simulink model "ThreephaseInverterWithoutLCfilter"  (R2024a)
settings: Solver=VariableStepAuto  StartTime=0.0  StopTime=.1  RelTol=1e-3
libraries: spsIGBTDiodeLib x6, simulink x3, spsVoltageMeasurementLib x3, spsDCVoltageSourceLib x1, spsGroundLib x1, spsSawtoothGeneratorLib x1, spsTHDLib x1, spsThreePhaseParallelRLCBranchLib x1, spsThreePhaseVIMeasurementLib x1, spspowerguiLib x1
settings Model: Creator=farza  LastModifiedBy=farza
settings DataIOCC: ReturnWorkspaceOutputs=off

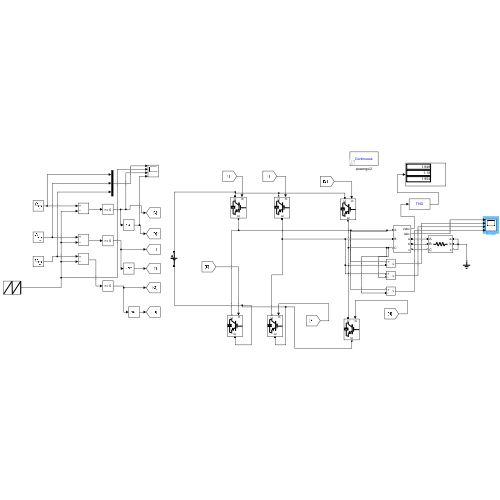
[thumbnail: Simulink's stored preview of the top-level diagram]
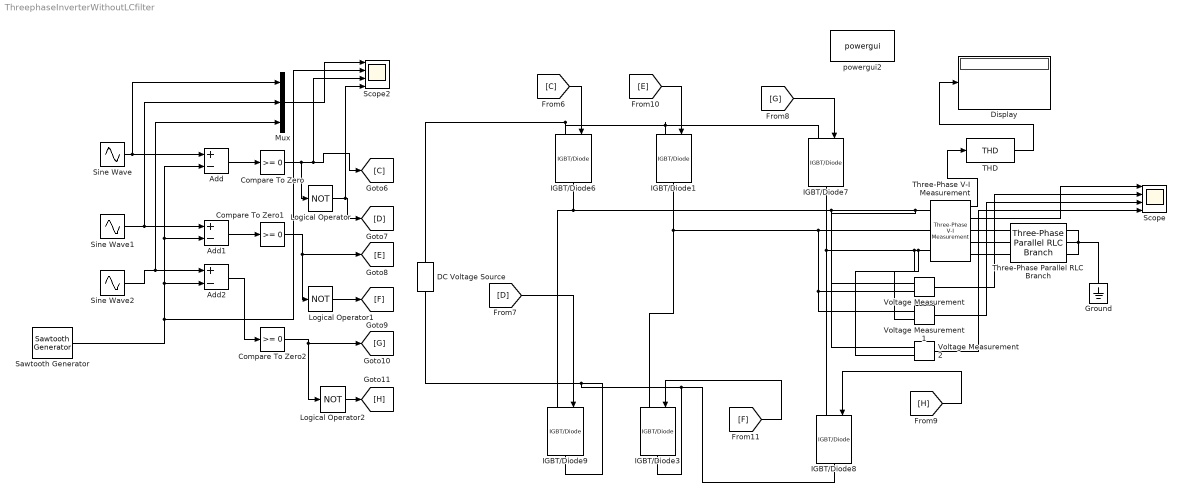
== system ThreephaseInverterWithoutLCfilter ==
  Add : Sum  Inputs=+-
  Add1 : Sum  Inputs=+-
  Add2 : Sum  Inputs=+-
  Compare To Zero : simulink/Logic and Bit Operations/Compare To Zero  relop=>=  OutDataTypeStr=boolean
  Compare To Zero1 : simulink/Logic and Bit Operations/Compare To Zero  relop=>=  OutDataTypeStr=boolean
  Compare To Zero2 : simulink/Logic and Bit Operations/Compare To Zero  relop=>=  OutDataTypeStr=boolean
  DC Voltage Source : spsDCVoltageSourceLib/DC Voltage Source  Amplitude=600  Measurements=None
  Display : Display
  Ground : spsGroundLib/Ground  LConnTagsString=a
  IGBT/Diode{1,3,6..9} (6 alike) : spsIGBTDiodeLib/IGBT//Diode  Ron=1e-3  Rs=1e5  Cs=inf  Measurements=off
  Logical Operator : Logic  Operator=NOT  AllPortsSameDT=off  OutDataTypeStr=boolean
  Logical Operator1 : Logic  Operator=NOT  AllPortsSameDT=off  OutDataTypeStr=boolean
  Logical Operator2 : Logic  Operator=NOT  AllPortsSameDT=off  OutDataTypeStr=boolean
  Mux : Mux  Inputs=3
  Sawtooth Generator : spsSawtoothGeneratorLib/Sawtooth Generator  Freq=5000  Phase=0  Ts=0
  Scope : Scope  NumInputPorts=4
  Scope2 : Scope  NumInputPorts=4
  Sine Wave : Sin  Frequency=2*pi*50  SampleTime=0
  Sine Wave1 : Sin  Frequency=2*pi*50  Phase=120  SampleTime=0
  Sine Wave2 : Sin  Frequency=2*pi*50  Phase=-120  SampleTime=0
  THD : spsTHDLib/THD  Freq=60  Ts=0
  Three-Phase Parallel RLC Branch : spsThreePhaseParallelRLCBranchLib/Three-Phase Parallel RLC Branch  LConnTagsString=A|B|C  RConnTagsString=A|B|C  BranchType=R  Resistance=60  Inductance=1e-3  Capacitance=1e-6  Measurements=None
  Three-Phase V-I Measurement : spsThreePhaseVIMeasurementLib/Three-Phase V-I Measurement  VoltageMeasurement=phase-to-phase  SetLabelV=off  LabelV=Vabc  Vpu=off  VpuLL=off  CurrentMeasurement=yes  SetLabelI=off  LabelI=Iabc  Ipu=off  Pbase=100e6  Vbase=500e3  OutputType=Complex  PhasorSimulation=off  PSBequivalent=0
  Voltage Measurement : spsVoltageMeasurementLib/Voltage Measurement  PhasorSimulation=off  OutputType=Complex  PSBequivalent=0
  Voltage Measurement1 : spsVoltageMeasurementLib/Voltage Measurement  PhasorSimulation=off  OutputType=Complex  PSBequivalent=0
  Voltage Measurement2 : spsVoltageMeasurementLib/Voltage Measurement  PhasorSimulation=off  OutputType=Complex  PSBequivalent=0
  powergui2 : spspowerguiLib/powergui  Priority=1  SimulationMode=Continuous  SampleTime=50e-6  frequency=60  Iterations=50  frequencyindice=0  Pbase=100e6  ErrMax=1e-4  UnitsV=kV  UnitsW=MW  buscounter=0  FunctionMessages=off  echomessages=off  EnableUseOfTLC=off  CurrentSourceSwitches=off  DisableSnubberDevices=off  DisableRonSwitches=off  DisableVfSwitches=off  DisplayEquations=off  AutomaticDiscreteSolvers=off  SolverType=Tustin/Backward Euler (TBE)  Interpol=off  ExternalGateDelay=off  methode=off  Ts=100  x0status=blocks  SPID=on  SwTol=0  HookPort=off  NonlinearTolerance=0  nMaxIteration=15  ContinueOnMaxIteration=off  RestoreLinks=warning  ResistiveCurrentMeasurement=off  Frange=[0:2:500]  Ylog=off  Xlog=on  ShowGrid=off  save=off  variable=ZData  structure=0  ZoomFFT=off  StartTime=0.0  cycles=1  DisplayStyle=1  fundamental=60  FreqAxis=off  MaxFrequency=1000  frequencyindicesteady=1  RmsSteady=1  display=off
  wires:
  Add/1 -> Compare To Zero/1
  [D] -> IGBT/Diode9/1
  Sawtooth Generator/1 -> Scope2/2, Add2/2, Add/2, Add1/2
  Compare To Zero/1 -> Logical Operator/1, Scope2/3, [C]
  [F] -> IGBT/Diode3/1
  Add2/1 -> Compare To Zero2/1
  Compare To Zero1/1 -> Logical Operator1/1, [E]
  [E] -> IGBT/Diode1/1
  Compare To Zero2/1 -> Logical Operator2/1, [G]
  Mux/1 -> Scope2/1
  THD/1 -> Display/1
  [H] -> IGBT/Diode8/1
  [C] -> IGBT/Diode6/1
  [G] -> IGBT/Diode7/1
  Logical Operator/1 -> Scope2/4, [D]
  Sine Wave/1 -> Add/1, Mux/1
  Sine Wave1/1 -> Mux/2, Add1/1
  Logical Operator1/1 -> [F]
  Logical Operator2/1 -> [H]
  Three-Phase V-I Measurement/1 -> THD/1
  Sine Wave2/1 -> Mux/3, Add2/1
  Add1/1 -> Compare To Zero1/1
  Three-Phase V-I Measurement/2 -> Scope/1
  Voltage Measurement/1 -> Scope/2
  Voltage Measurement1/1 -> Scope/3
  Voltage Measurement2/1 -> Scope/4
  connections:
  IGBT/Diode6/LConn1 -- DC Voltage Source/RConn1 -- IGBT/Diode1/LConn1 -- IGBT/Diode7/LConn1
  Three-Phase Parallel RLC Branch/LConn3 -- Three-Phase V-I Measurement/RConn3
  Three-Phase Parallel RLC Branch/LConn2 -- Three-Phase V-I Measurement/RConn2
  IGBT/Diode6/RConn1 -- Voltage Measurement2/LConn1 -- Voltage Measurement/LConn1 -- Three-Phase V-I Measurement/LConn1 -- IGBT/Diode9/LConn1
  IGBT/Diode3/LConn1 -- Voltage Measurement1/LConn1 -- Voltage Measurement/LConn2 -- Three-Phase V-I Measurement/LConn2 -- IGBT/Diode1/RConn1
  IGBT/Diode7/RConn1 -- IGBT/Diode8/LConn1 -- Voltage Measurement1/LConn2 -- Voltage Measurement2/LConn2 -- Three-Phase V-I Measurement/LConn3
  IGBT/Diode8/RConn1 -- DC Voltage Source/LConn1 -- IGBT/Diode9/RConn1 -- IGBT/Diode3/RConn1
  Three-Phase Parallel RLC Branch/LConn1 -- Three-Phase V-I Measurement/RConn1
  Three-Phase Parallel RLC Branch/RConn3 -- Three-Phase Parallel RLC Branch/RConn1 -- Ground/LConn1 -- Three-Phase Parallel RLC Branch/RConn2
